simulink model "ASML_Tune"  (R2022a)
settings: Solver=FixedStepAuto  StartTime=0.0  StopTime=1  FixedStep=Ts  RelTol=1e-3
model workspace (MAT data in the model file):
  InitRf = 0.627718676731
  enab = 1
  eol = 6
  euvTarget = Simulink.Parameter
  euvTarget.Value = 4.4
  euvTarget.DataType = 'auto'
  euvTarget.Complexity = 'real'
  euvTarget.Dimensions = [1 1]
undefined symbols (not defined in the file): Ts
libraries: simulink x1
settings Model: Creator=rjacques  LastModifiedBy=maxcr
settings SolverCC: AlgebraicLoopSolver=TrustRegion
settings DataIOCC: ExternalInput=extInput_SimulateEuvControl  DSMLogging=off  SaveTime=off  ReturnWorkspaceOutputs=off
settings OptimizationCC: EfficientMapNaN2IntZero=off
settings DebuggingCC: AlgebraicLoopMsg=none  UnconnectedInputMsg=warning  UnconnectedOutputMsg=warning  UnconnectedLineMsg=warning  SFMachineParentedDataDiag=warning  ArithmeticOperatorsInVariantConditions=warning
settings HardwareCC: TargetBitPerPointer=64  TargetBitPerSizeT=64  TargetBitPerPtrDiffT=64  TargetLongLongMode=on  TargetIntDivRoundTo=Zero  TargetEndianess=LittleEndian  TargetWordSize=64  TargetHWDeviceType=MATLAB Host  ProdEqTarget=off
settings SFSimCC: SimUseLocalCustomCode=off  CustomCodeUndefinedFunction=UseInterfaceOnly
settings RTWCC: SystemTargetFile=accel.tlc  TemplateMakefile=accel_default_tmf  RTWVerbose=off  DLArmComputeVersion=19.05
settings CodeAppCC: MaxIdLength=128
settings STFCustomTargetCC: ConcurrentExecutionCompliant=on  MATLABClassNameForMDSCustomization=Simulink.SoftwareTarget.TargetSpecificTriggerConfigurationBase  SystemTargetFile=accel.tlc

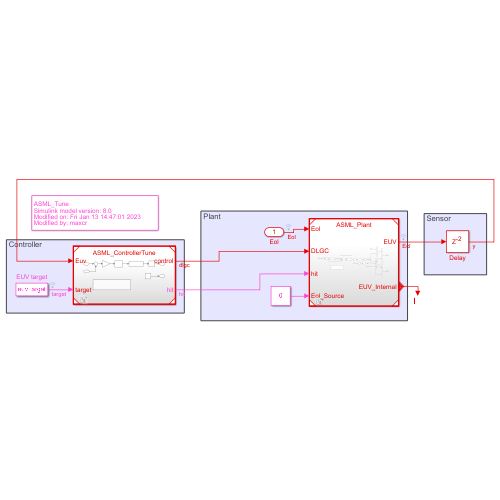
[thumbnail: Simulink's stored preview of the top-level diagram]
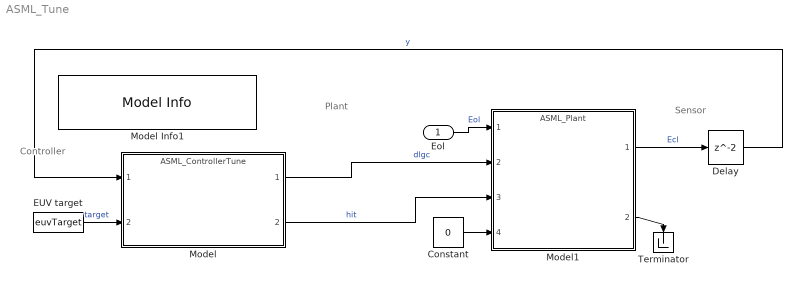
== system ASML_Tune ==
  note: Sensor
  note: Controller
  note: Plant
  Eol : Inport  OutDataTypeStr=double  SampleTime=Ts
  Constant : Constant  Value=0
  Delay : Delay  InitialCondition=5
  EUV target : Constant  Value=euvTarget  OutDataTypeStr=double
  Model : ModelReference  ModelNameDialog=ASML_ControllerTune.slx  SimulationMode=Normal  ModelReferenceVersion=5.29
  Model Info1 : simulink/Model-Wide Utilities/Model Info  Frame=on  DisplayStringWithTags=|  HorizontalTextAlignment=Left  LeftAlignmentValue=0.02
      | %<ModelName>
      | Simulink model version: %<ModelVersion>
      | Modified on: %<LastModificationDate>
      | Modified by: %<ModifiedBy>
  Model1 : ModelReference  ModelNameDialog=ASML_Plant.slx  SimulationMode=Normal  ModelReferenceVersion=8.5
  Terminator : Terminator
  wires:
  EUV target/1 -> Model/2  "target"
  Eol/1 -> Model1/1  "Eol"
  Delay/1 -> Model/1  "y"
  Model/1 -> Model1/2  "dlgc"
  Model/2 -> Model1/3  "hit"
  Model1/1 -> Delay/1  "Ecl"
  Model1/2 -> Terminator/1
  Constant/1 -> Model1/4
